simulink model "swing_up_energy_2"  (R2019b)
settings: Solver=VariableStepAuto  StartTime=0.0  StopTime=6  RelTol=1e-3
undefined symbols (not defined in the file): Klqi_int, Klqi_state, Parameters
settings Model: Creator=Samsung  LastModifiedBy=pietr
settings SolverCC: ZeroCrossAlgorithm=Adaptive
settings DebuggingCC: IgnoredZcDiagnostic=none

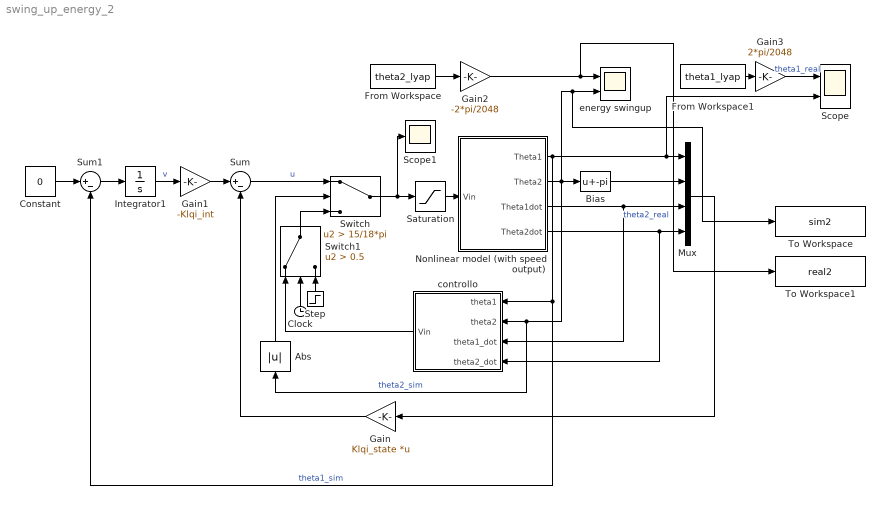
== system swing_up_energy_2 ==
  Abs : Abs  ZeroCross=off
  Bias : Bias  Bias=-pi
  Clock : Clock
  Constant : Constant  Value=0
  From Workspace : FromWorkspace  VariableName=theta2_lyap  SampleTime=0
  From Workspace1 : FromWorkspace  VariableName=theta1_lyap  SampleTime=0
  Gain : Gain  Gain=Klqi_state  Multiplication=Matrix(K*u)
  Gain1 : Gain  Gain=-Klqi_int
  Gain2 : Gain  Gain=-2*pi/2048
  Gain3 : Gain  Gain=2*pi/2048
  Integrator1 : Integrator
  Mux : Mux
  Nonlinear model (with speed output) : Subsystem
  Saturation : Saturate  UpperLimit=10  LowerLimit=-10  ZeroCross=off
  Scope : Scope  NumInputPorts=2
  Scope1 : Scope
  Step : Step  Time=0.1  After=-1  SampleTime=0
  Sum : Sum  Inputs=|+-
  Sum1 : Sum  Inputs=|+-
  Switch : Switch  Criteria=u2 > Threshold  Threshold=15/18*pi
  Switch1 : Switch  Criteria=u2 > Threshold  Threshold=0.5
  To Workspace : ToWorkspace  VariableName=sim2  SampleTime=-1
      settings: Save2DSignal=2-D array (concatenate along first dimension)
  To Workspace1 : ToWorkspace  VariableName=real2  SampleTime=-1
      settings: Save2DSignal=2-D array (concatenate along first dimension)
  controllo : Subsystem
  energy swingup : Scope  NumInputPorts=2
  wires:
  Sum1/1 -> Integrator1/1
  Mux/1 -> Gain/1
  Nonlinear model (with speed output)/1(Theta1) -> Scope/2, Mux/1, controllo/1(theta1), Sum1/2  "theta1_sim"
  Saturation/1 -> Nonlinear model (with speed output)/1(Vin)
  Bias/1 -> Mux/2
  Integrator1/1 -> Gain1/1  "v"
  Gain1/1 -> Sum/1
  Nonlinear model (with speed output)/4(Theta2dot) -> controllo/4(theta2_dot), Mux/4
  Gain/1 -> Sum/2
  Nonlinear model (with speed output)/2(Theta2) -> To Workspace/1, energy swingup/2, Abs/1, controllo/2(theta2), Bias/1  "theta2_sim"
  Constant/1 -> Sum1/1
  Sum/1 -> Switch/1  "u"
  Abs/1 -> Switch/2
  Switch/1 -> Scope1/1, Saturation/1
  controllo/1(Vin) -> Switch1/1
  Switch1/1 -> Switch/3
  Clock/1 -> Switch1/2
  Step/1 -> Switch1/3
  Nonlinear model (with speed output)/3(Theta1dot) -> controllo/3(theta1_dot), Mux/3
  From Workspace/1 -> Gain2/1
  Gain2/1 -> To Workspace1/1, energy swingup/1  "theta2_real"
  From Workspace1/1 -> Gain3/1
  Gain3/1 -> Scope/1  "theta1_real"

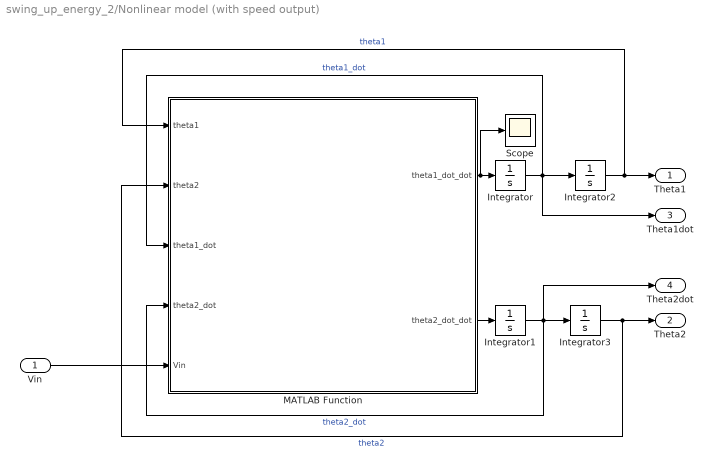
== system swing_up_energy_2/Nonlinear model (with speed output) ==
  Vin : Inport
  Integrator{,1..3} (4 alike) : Integrator
  MATLAB Function : MATLAB Function  TreatAsAtomicUnit=on  mask{Pars=Parameters}
      mask prompts: Pars "Struct containing model parameters"
  Scope : Scope
  Theta1 : Outport
  Theta2 : Outport  Port=2
  Theta1dot : Outport  Port=3
  Theta2dot : Outport  Port=4
  wires:
  Integrator/1 -> Theta1dot/1, MATLAB Function/3(theta1_dot), Integrator2/1  "theta1_dot"
  Integrator1/1 -> Theta2dot/1, MATLAB Function/4(theta2_dot), Integrator3/1  "theta2_dot"
  MATLAB Function/1(theta1_dot_dot) -> Scope/1, Integrator/1
  Integrator3/1 -> Theta2/1, MATLAB Function/2(theta2)  "theta2"
  MATLAB Function/2(theta2_dot_dot) -> Integrator1/1
  Integrator2/1 -> MATLAB Function/1(theta1), Theta1/1  "theta1"
  Vin/1 -> MATLAB Function/5(Vin)

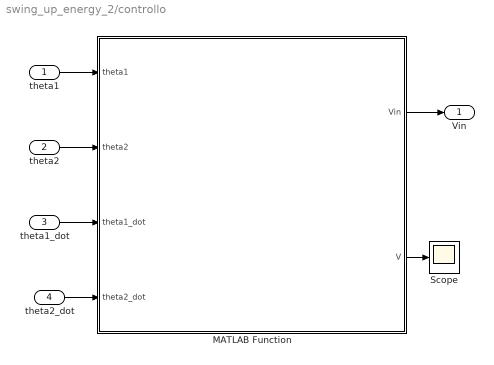
== system swing_up_energy_2/controllo ==
  theta1 : Inport
  theta2 : Inport  Port=2
  theta1_dot : Inport  Port=3
  theta2_dot : Inport  Port=4
  MATLAB Function : MATLAB Function  TreatAsAtomicUnit=on  mask{Pars=Parameters}
      mask prompts: Pars "Struct containing model parameters"
  Scope : Scope
  Vin : Outport
  wires:
  MATLAB Function/1(Vin) -> Vin/1
  theta1/1 -> MATLAB Function/1(theta1)
  theta2/1 -> MATLAB Function/2(theta2)
  theta1_dot/1 -> MATLAB Function/3(theta1_dot)
  theta2_dot/1 -> MATLAB Function/4(theta2_dot)
  MATLAB Function/2(V) -> Scope/1

== matlab function swing_up_energy_2/controllo/MATLAB Function ==
  data: theta1 input size=1; Vin output size=1; theta2 input size=1; theta1_dot input size=1; theta2_dot input size=1; Pars parameter; V output
function [Vin, V]  = fcn(theta1, theta2, theta1_dot, theta2_dot, Pars)
   const = 1000*1;
   k1 = Pars.Jeq + Pars.m2*(Pars.l1^2 + Pars.x2^2*sin(theta2)^2);
   k2 = Pars.m2*Pars.l1*Pars.x2*cos(theta2);
   % attenzione k3 diverso da funzione modello non lineare 
   k3 = 2*Pars.m2*Pars.x2^2*sin(theta2)*cos(theta2)*theta1_dot*theta2_dot - Pars.m2*Pars.l1*Pars.x2*sin(theta2)*theta2_dot^2 +Pars.Ks*theta1 + (Pars.Km^2)/Pars.Rm*theta1_dot + Pars.Kf1*theta1_dot;
   k4 = Pars.m2*Pars.l1*Pars.x2*cos(theta2);
   k5 = Pars.m2*Pars.x2^2 + Pars.I2;
   k6 = - Pars.m2*Pars.x2^2*sin(theta2)*cos(theta2)*theta1_dot^2 + Pars.m2*Pars.g*Pars.x2*sin(theta2) + Pars.Kf2*theta2_dot;
   
   % energia = energia cinetica + energia potenziale (prendo come 0 down)
   E = 1/2*(Pars.I2+Pars.m2*Pars.x2^2)*theta2_dot^2 + Pars.m2*Pars.g*(Pars.x2-Pars.x2*cos(theta2));
   Eup = Pars.m2*Pars.g*(Pars.x2+Pars.x2)*1.08; %aumento un po' Eup per attrito
   
   % funzione di Lyapunov V>0
   V = 1/2*(E-Eup)^2;
   
   % derivata lyapunov Vdot
   %Vdot = (E-Eup)*theta2_dot*((Pars.I2+Pars.m2*Pars.x2^2)*theta2_dot_dot+Pars.m2*Pars.g*Pars.x2*sin(theta2));
   
   % impongo theta2dotdot tale che derivata di V <0
   theta2_dot_dot = -Pars.m2*Pars.g*Pars.x2*sin(theta2)/(Pars.I2+Pars.m2*Pars.x2^2) -const*(E-Eup)*sign(theta2_dot);
   
   % calcolo Vin in base a modello non lineare
   Vin = (k4*k3-k1*k6-theta2_dot_dot*(k1*k5-k2*k4))*Pars.Rm/Pars.Km/k4;
   
end

== matlab function swing_up_energy_2/Nonlinear model (with speed output)/MATLAB Function ==
  data: theta1 input size=1; theta1_dot_dot output size=1; theta2 input size=1; theta1_dot input size=1; theta2_dot input size=1; Vin input size=1; theta2_dot_dot output size=1; Pars parameter
function [theta1_dot_dot,theta2_dot_dot] = fcn(theta1, theta2, theta1_dot, theta2_dot,Vin, Pars)

   k1 = Pars.Jeq + Pars.m2*(Pars.l1^2 + Pars.x2^2*sin(theta2)^2);
   k2 = Pars.m2*Pars.l1*Pars.x2*cos(theta2);
   k3 = 2*Pars.m2*Pars.x2^2*sin(theta2)*cos(theta2)*theta1_dot*theta2_dot - Pars.m2*Pars.l1*Pars.x2*sin(theta2)*theta2_dot^2 +Pars.Ks*theta1 - Pars.Km/Pars.Rm*Vin + (Pars.Km^2)/Pars.Rm*theta1_dot + Pars.Kf1*theta1_dot;
   k4 = Pars.m2*Pars.l1*Pars.x2*cos(theta2);
   k5 = Pars.m2*Pars.x2^2 + Pars.I2;
   k6 = - Pars.m2*Pars.x2^2*sin(theta2)*cos(theta2)*theta1_dot^2 + Pars.m2*Pars.g*Pars.x2*sin(theta2) + Pars.Kf2*theta2_dot;


theta1_dot_dot = (k2*k6 - k3*k5)/(k1*k5 - k2*k4);
theta2_dot_dot = -(k1*k6 - k3*k4)/(k1*k5 - k2*k4);
